simulink model "WS_17_Nils_Bestehorn_modell"  (R2021b)
settings: Solver=FixedStepAuto  StartTime=0.0  StopTime=20  FixedStep=0.01  RelTol=1e-3
values from neighbouring files (symbols this model uses):
  c1 = 120*(1/10^-3)    (= 120000)    [WS_17_Nils_Bestehorn_mfile.m]
  c2 = 20*(1/10^-3)    (= 20000)    [WS_17_Nils_Bestehorn_mfile.m]
  cp = 0.5*(1/10^-3)    (= 500)    [WS_17_Nils_Bestehorn_mfile.m]
  d2 = 0.5*(1/10^-3)    (= 500)    [WS_17_Nils_Bestehorn_mfile.m]
  dp = 0.1*(1/10^-3)    (= 100)    [WS_17_Nils_Bestehorn_mfile.m]
  m1 = 30    [WS_17_Nils_Bestehorn_mfile.m]
  m2 = 250    [WS_17_Nils_Bestehorn_mfile.m]
  zh = 10*10^-2    (= 0.1)    [WS_17_Nils_Bestehorn_mfile.m]
undefined symbols (not defined in the file or in its folder): sigbuilder_block
libraries: simulink x1
settings Model: Creator=nilsb  LastModifiedBy=nilsb

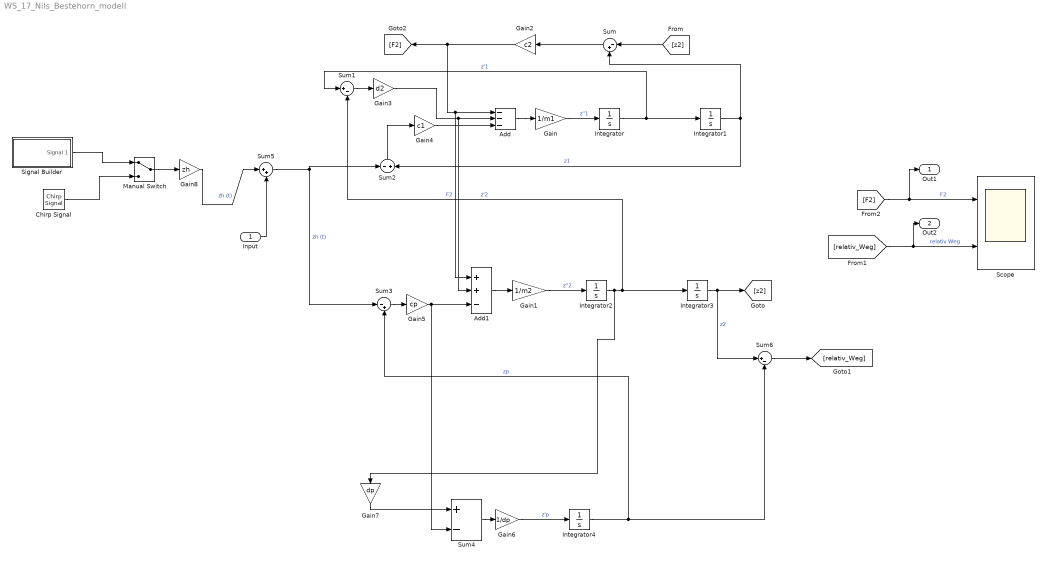
== system WS_17_Nils_Bestehorn_modell ==
  Input : Inport
  Add : Sum  Inputs=---
  Add1 : Sum  Inputs=++-
  Chirp Signal : simulink/Sources/Chirp Signal  f1=0.01  T=20  f2=20
  Gain : Gain  Gain=1/m1
  Gain1 : Gain  Gain=1/m2
  Gain2 : Gain  Gain=c2
  Gain3 : Gain  Gain=d2
  Gain4 : Gain  Gain=c1
  Gain5 : Gain  Gain=cp
  Gain6 : Gain  Gain=1/dp
  Gain7 : Gain  Gain=dp
  Gain8 : Gain  Gain=zh
  Integrator{,1..4} (5 alike) : Integrator
  Manual Switch : ManualSwitch
  Scope : Scope  NumInputPorts=2
  Signal Builder : Subsystem  Tag=STV Subsys  LoadFcn=sigbuilder_block('load');  StartFcn=sigbuilder_block('start');  StopFcn=sigbuilder_block('stop');  ClipboardFcn=sigbuilder_block('clipboard');  mask(Sigbuilder block){tuvar=[0:10]}
      mask help: Simulink:masks:SigbuilderBlock_MD
      mask init:
      | if ~strcmp(get_param(bdroot(gcbh),'SimulationStatus'),'stopped') tuvar = sigbuilder_block('maskInit'); end
      settings: CopyFcn=sigbuilder_block('copy');  DeleteFcn=sigbuilder_block('delete');  ModelCloseFcn=sigbuilder_block('modelClose');  PreSaveFcn=sigbuilder_block('preSave');  PauseFcn=sigbuilder_block('pause');  ContinueFcn=sigbuilder_block('continue');  NameChangeFcn=sigbuilder_block('namechange');  OpenFcn=sigbuilder_block('open',[437.6 199.2 550.4 400 ]);  CloseFcn=sigbuilder_block('close');
      mask Display: plot(0, 0, 100, 100,[2, 2, 32, 32, 2], [68, 8, 8, 68, 68],[32, 2], [38, 38], [32, 19, 2],[53, 60, 44], [32, 17, 17, 2],[16, 16, 31, 31]);txt = getActiveGroup(gcbh);text(2, 100, txt,'verticalAlignment', 'top');
  Sum : Sum  Inputs=|-+
  Sum1 : Sum  Inputs=|+-
  Sum2 : Sum  Inputs=-+
  Sum3 : Sum  Inputs=|-+
  Sum4 : Sum  Inputs=+-
  Sum5 : Sum  Inputs=|++
  Sum6 : Sum  Inputs=|+-
  Out1 : Outport
  Out2 : Outport  Port=2
  wires:
  Integrator/1 -> Sum1/1, Integrator1/1  "z'1"
  Gain/1 -> Integrator/1  "z''1"
  Integrator1/1 -> Sum2/2, Sum/2  "z1"
  Integrator2/1 -> Integrator3/1, Sum1/2, Gain7/1  "z'2"
  Integrator3/1 -> Sum6/1, [z2]  "z2"
  Gain1/1 -> Integrator2/1  "z''2"
  Add/1 -> Gain/1
  Add1/1 -> Gain1/1
  Sum/1 -> Gain2/1
  [z2] -> Sum/1
  Gain4/1 -> Add/3
  Sum1/1 -> Gain3/1
  Sum2/1 -> Gain4/1
  Gain8/1 -> Sum5/1  "zh (t)"
  Gain2/1 -> [F2], Add1/1, Add/1  "F2"
  Gain3/1 -> Add1/2, Add/2
  Integrator4/1 -> Sum6/2, Sum3/2  "zp"
  Sum3/1 -> Gain5/1
  Gain6/1 -> Integrator4/1  "z'p"
  Sum4/1 -> Gain6/1
  Gain7/1 -> Sum4/1
  Gain5/1 -> Add1/3, Sum4/2
  Manual Switch/1 -> Gain8/1
  Chirp Signal/1 -> Manual Switch/2
  Signal Builder/1(Signal 1) -> Manual Switch/1
  Sum5/1 -> Sum3/1, Sum2/1  "zh (t)"
  Input/1 -> Sum5/2
  [F2] -> Out1/1, Scope/1  "F2"
  [relativ_Weg] -> Out2/1, Scope/2  "relativ Weg"
  Sum6/1 -> [relativ_Weg]

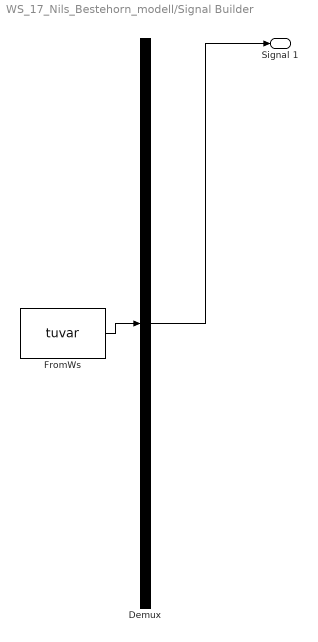
== system WS_17_Nils_Bestehorn_modell/Signal Builder ==
  Demux : Demux  Tag=STV Demux  Outputs=1
      settings: DisplayOption=none
  FromWs : FromWorkspace  Tag=STV FromWs  VariableName=tuvar
      SigBuilderData=|
      | common.afterFinalStr = 'Extrapolate'
      | common.sampleTime = 0
      | dataSet.timeRange = [0 4]
      | dataSet.name = 'Group 1'
      | sbobj.Groups.Name = 'Group 1'
      | sbobj.Groups.Signals.Name = 'Signal 1'
      | sbobj.Groups.Signals.XData = [0 0.25 1.9 2 4]
      | sbobj.Groups.Signals.YData = [0 1 1 0 0]
      | sbobj.Groups.TimeRange = [0 4]
  Signal 1 : Outport  Tag=STV Outport
  wires:
  Demux/1 -> Signal 1/1
  FromWs/1 -> Demux/1
